simulink model "untitled"  (R2018a)
settings: Solver=FixedStepAuto  StartTime=2  StopTime=5  RelTol=1e-3
libraries: powerlib x14
settings Model: Creator=Ali  LastModifiedBy=Ali

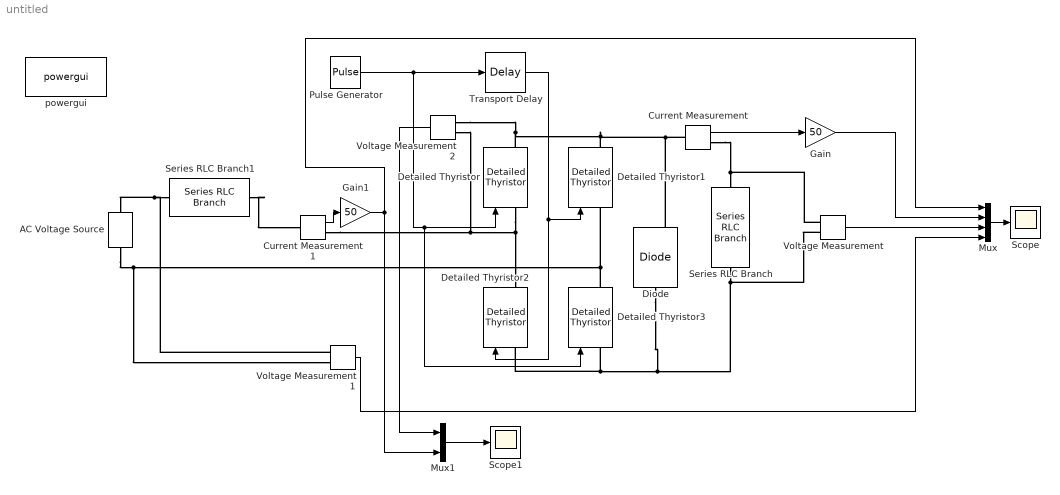
== system untitled ==
  AC Voltage Source : powerlib/Electrical Sources/AC Voltage Source  Amplitude=200  Phase=0  Frequency=50  SampleTime=0  Measurements=None  BusType=swing  Pref=10e3  Qref=0  Qmin=-inf  Qmax=+inf
  Current Measurement : powerlib/Measurements/Current Measurement  PhasorSimulation=off  OutputType=Complex  PSBequivalent=0
  Current Measurement1 : powerlib/Measurements/Current Measurement  PhasorSimulation=off  OutputType=Complex  PSBequivalent=0
  Detailed Thyristor{,1..3} (4 alike) : powerlib/Power Electronics/Detailed Thyristor  Ron=0.001  Lon=1e-3  Vf=0.8  IL=0.1  Tq=100e-6  IC=0  Rs=500  Cs=250e-9  Measurements=on
      settings: SourceProductName=Simscape Power Systems  SourceProductBaseCode=PS
  Diode : powerlib/Power Electronics/Diode  Ron=0.001  Lon=0  Vf=0.8  IC=0  UseSnubber=0  Rs=500  Cs=250e-9  Measurements=on
  Gain : Gain  Gain=50
  Gain1 : Gain  Gain=50
  Mux : Mux
  Mux1 : Mux  Inputs=2
  Pulse Generator : DiscretePulseGenerator  PulseType=Time based  Amplitude=5  Period=0.02  PulseWidth=5  PhaseDelay=(60*0.02)/360
  Scope : Scope
  Scope1 : Scope
  Series RLC Branch : powerlib/Elements/Series RLC Branch  LConnTagsString=__new0  RConnTagsString=__new0  BranchType=RL  Resistance=24  Inductance=0.4575  SetiL0=off  InitialCurrent=0  Capacitance=1e-6  Setx0=off  InitialVoltage=0  Measurements=None
  Series RLC Branch1 : powerlib/Elements/Series RLC Branch  LConnTagsString=__new0  RConnTagsString=__new0  BranchType=L  Resistance=24  Inductance=0.005  SetiL0=off  InitialCurrent=0  Capacitance=1e-6  Setx0=off  InitialVoltage=0  Measurements=None
  Transport Delay : TransportDelay  DelayTime=0.01
  Voltage Measurement : powerlib/Measurements/Voltage Measurement  PhasorSimulation=off  OutputType=Complex  PSBequivalent=0
  Voltage Measurement1 : powerlib/Measurements/Voltage Measurement  PhasorSimulation=off  OutputType=Complex  PSBequivalent=0
  Voltage Measurement2 : powerlib/Measurements/Voltage Measurement  PhasorSimulation=off  OutputType=Complex  PSBequivalent=0
  powergui : powerlib/powergui  Priority=1  SimulationMode=Discrete  SampleTime=50e-6  frequency=60  Iterations=50  frequencyindice=50  Pbase=100e6  ErrMax=1e-4  UnitsV=kV  UnitsW=MW  buscounter=0  FunctionMessages=off  echomessages=off  EnableUseOfTLC=off  CurrentSourceSwitches=off  DisableSnubberDevices=off  DisableRonSwitches=off  DisableVfSwitches=off  DisplayEquations=off  SolverType=Tustin/Backward Euler (TBE)  Interpol=off  ExternalGateDelay=off  methode=off  Ts=100  x0status=blocks  SPID=off  SwTol=0  HookPort=off  RestoreLinks=warning  ResistiveCurrentMeasurement=off  Frange=[0:2:500]  Ylog=off  Xlog=on  ShowGrid=off  save=off  variable=ZData  structure=0  ZoomFFT=off  StartTime=0.0  cycles=1  DisplayStyle=1  fundamental=60  FreqAxis=off  MaxFrequency=1000  frequencyindicesteady=1  RmsSteady=1  display=off
  wires:
  Mux/1 -> Scope/1
  Current Measurement/1 -> Gain/1
  Voltage Measurement/1 -> Mux/3
  Voltage Measurement1/1 -> Mux/4
  Gain/1 -> Mux/2
  Gain1/1 -> Mux1/2, Mux/1
  Transport Delay/1 -> Detailed Thyristor2/1, Detailed Thyristor1/1
  Pulse Generator/1 -> Detailed Thyristor/1, Detailed Thyristor3/1, Transport Delay/1
  Mux1/1 -> Scope1/1
  Voltage Measurement2/1 -> Mux1/1
  Current Measurement1/1 -> Gain1/1
  connections:
  Voltage Measurement/LConn1 -- Current Measurement/RConn1 -- Series RLC Branch/LConn1
  Detailed Thyristor2/LConn1 -- Detailed Thyristor3/LConn1 -- Diode/LConn1 -- Voltage Measurement/LConn2 -- Series RLC Branch/RConn1
  Detailed Thyristor/RConn1 -- Diode/RConn1 -- Current Measurement/LConn1 -- Detailed Thyristor1/RConn1 -- Voltage Measurement2/LConn2
  Voltage Measurement1/LConn1 -- Series RLC Branch1/RConn1 -- AC Voltage Source/RConn1
  AC Voltage Source/LConn1 -- Detailed Thyristor1/LConn1 -- Detailed Thyristor3/RConn1 -- Voltage Measurement1/LConn2
  Detailed Thyristor/LConn1 -- Voltage Measurement2/LConn1 -- Current Measurement1/RConn1 -- Detailed Thyristor2/RConn1
  Series RLC Branch1/LConn1 -- Current Measurement1/LConn1
